simulink model "sub_1"  (Simulink 9.2)
settings: Solver=ode45  StartTime=0.0  StopTime=3  RelTol=1e-3  EnableMultiTasking=on
settings Model: Creator=student  LastModifiedBy=murad
settings OptimizationCC: ExpressionDepthLimit=2147483647
settings DebuggingCC: SolverPrmCheckMsg=warning

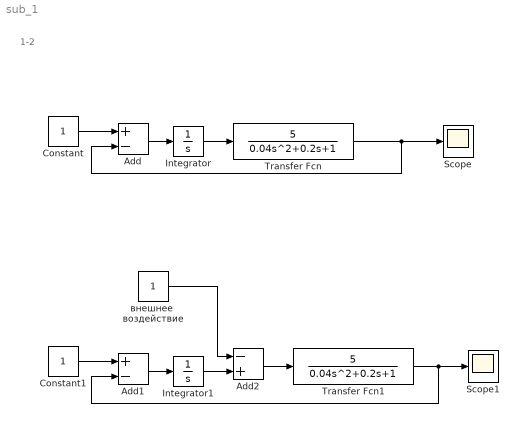
== system sub_1 ==
  note: 1-2
  Add : Sum  Inputs=+-
  Add1 : Sum  Inputs=+-
  Add2 : Sum  Inputs=-+
  Constant : Constant
  Constant1 : Constant
  Integrator : Integrator
  Integrator1 : Integrator
  Scope : Scope
  Scope1 : Scope
  Transfer Fcn : TransferFcn  Numerator=[5]  Denominator=[0.04 0.2 1]
  Transfer Fcn1 : TransferFcn  Numerator=[5]  Denominator=[0.04 0.2 1]
  внешнее  воздействие : Constant
  wires:
  Constant/1 -> Add/1
  Transfer Fcn/1 -> Add/2, Scope/1
  Add/1 -> Integrator/1
  Integrator/1 -> Transfer Fcn/1
  Add1/1 -> Integrator1/1
  Transfer Fcn1/1 -> Add1/2, Scope1/1
  Constant1/1 -> Add1/1
  Integrator1/1 -> Add2/2
  Add2/1 -> Transfer Fcn1/1
  внешнее  воздействие/1 -> Add2/1
